simulink model "diff_drive_tracking_new"  (R2019b)
settings: Solver=ode45  StartTime=0.0  StopTime=T  MaxStep=0.01  RelTol=1e-3  EnableMultiTasking=on
values from neighbouring files (symbols this model uses):
  b = 1    [init.m]
  distc = 14.5    [init.m]
  radius = 3.25    [init.m]
  theta_0 = 0    [init.m]
  x_0 = 10    [init.m]
  y_0 = 40    [init.m]
undefined symbols (not defined in the file or in its folder): diff_drive, localization, potential
settings Model: ExtModeAutoUpdateStatusClock=off  Creator=marilena  LastModifiedBy=adelina
settings DataIOCC: LimitDataPoints=on  SaveFormat=Array  SignalLoggingSaveFormat=ModelDataLogs  ReturnWorkspaceOutputs=off
settings OptimizationCC: ExpressionDepthLimit=2147483647  LifeSpan=inf
settings DebuggingCC: SaveWithParameterizedLinksMsg=none  UnderspecifiedInitializationDetection=Classic  MergeDetectMultiDrivingBlocksExec=none  SolverPrmCheckMsg=warning  FcnCallInpInsideContextMsg=warning  StateNameClashWarn=warning  SFUnexpectedBacktrackingDiag=warning  SFNoUnconditionalDefaultTransitionDiag=warning  ArithmeticOperatorsInVariantConditions=warning
settings HardwareCC: ProdBitPerPointer=32  ProdBitPerSizeT=32  ProdBitPerPtrDiffT=32  ProdLargestAtomicFloat=None  ProdIntDivRoundTo=Undefined  ProdEndianess=Unspecified  ProdWordSize=32  ProdHWDeviceType=32-bit Generic  TargetHWDeviceType=32-bit Generic
settings ModelReferenceCC: PropagateSignalLabelsOutOfModel=off
settings SFSimCC: SimUseLocalCustomCode=off  CustomCodeUndefinedFunction=UseInterfaceOnly
settings RTWCC: RTWUseLocalCustomCode=off
settings CodeAppCC: StateflowObjectComments=on
settings GRTTargetCC: TargetFcnLib=ansi_tfl_tmw.mat  TargetLangStandard=C89/C90 (ANSI)  CombineOutputUpdateFcns=off  GRTInterface=on
settings ConfigComp: CovMetricSettings=dw  CovHtmlReporting=on  CovSaveCumulativeToWorkspaceVar=on  CovSaveSingleToWorkspaceVar=on  CovExternalEMLEnable=off

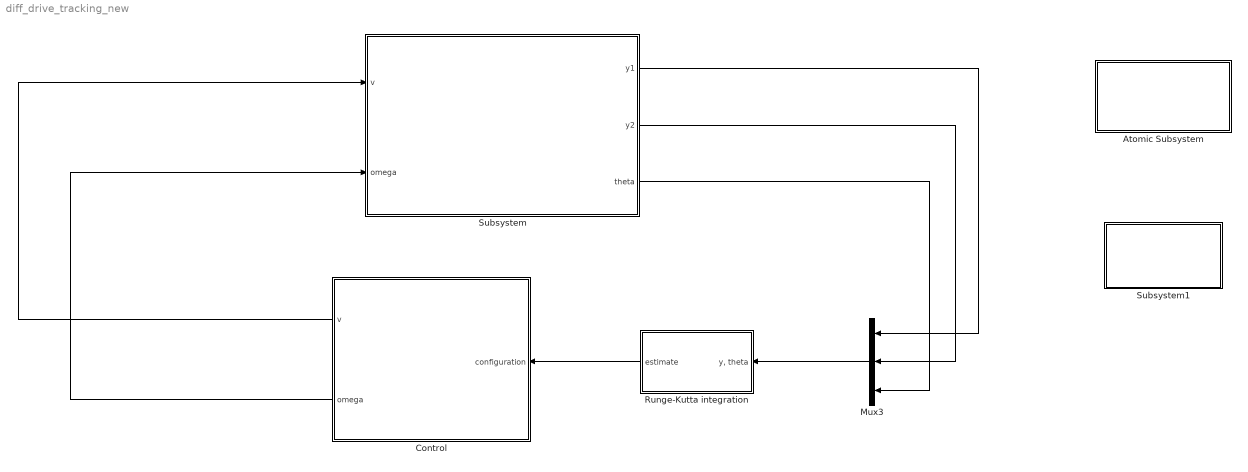
== system diff_drive_tracking_new ==
  Atomic Subsystem : Subsystem  TreatAsAtomicUnit=on
      settings: OpenFcn=init
      mask Display: disp('initialization')
  Control : Subsystem
  Mux3 : Mux  Inputs=3
  Runge-Kutta integration : Subsystem
  Subsystem : Subsystem
  Subsystem1 : Subsystem
      settings: OpenFcn=plots
      mask Display: disp('plots')
  wires:
  Mux3/1 -> Runge-Kutta integration/1("y, theta")
  Control/1(v) -> Subsystem/1(v)
  Control/2(omega) -> Subsystem/2(omega)
  Subsystem/1(y1) -> Mux3/1
  Subsystem/2(y2) -> Mux3/2
  Subsystem/3(theta) -> Mux3/3
  Runge-Kutta integration/1("estimate ") -> Control/1(configuration)

== system diff_drive_tracking_new/Atomic Subsystem ==

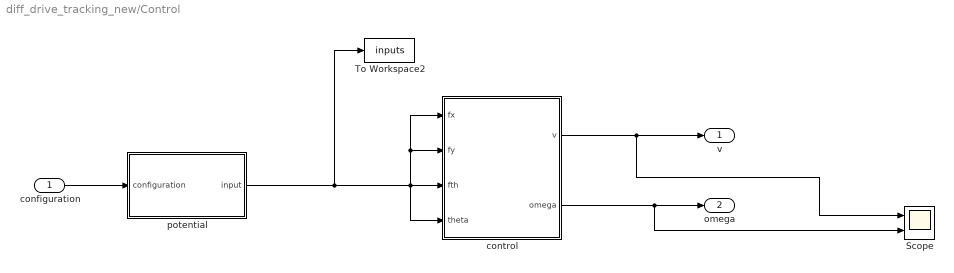
== system diff_drive_tracking_new/Control ==
  configuration : Inport
  Scope : Scope  NumInputPorts=2
  To Workspace2 : ToWorkspace  VariableName=inputs  SaveFormat=Structure With Time  SampleTime=-1
  control : Subsystem
  potential : Subsystem
  v : Outport
  omega : Outport  Port=2
  wires:
  control/2(omega) -> Scope/2, omega/1
  configuration/1 -> potential/1(configuration)
  potential/1(input) -> To Workspace2/1, control/1(fx), control/2(fy), control/4(theta), control/3(fth)
  control/1(v) -> Scope/1, v/1

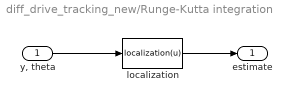
== system diff_drive_tracking_new/Runge-Kutta integration ==
  "y, theta" : Inport
  localization : MATLABFcn  Tag={'prova'}  Description=cartesian regulator  MATLABFcn=localization(u)  Output1D=off
  "estimate " : Outport  VectorParamsAs1DForOutWhenUnconnected=off
  wires:
  "y, theta"/1 -> localization/1
  localization/1 -> "estimate "/1

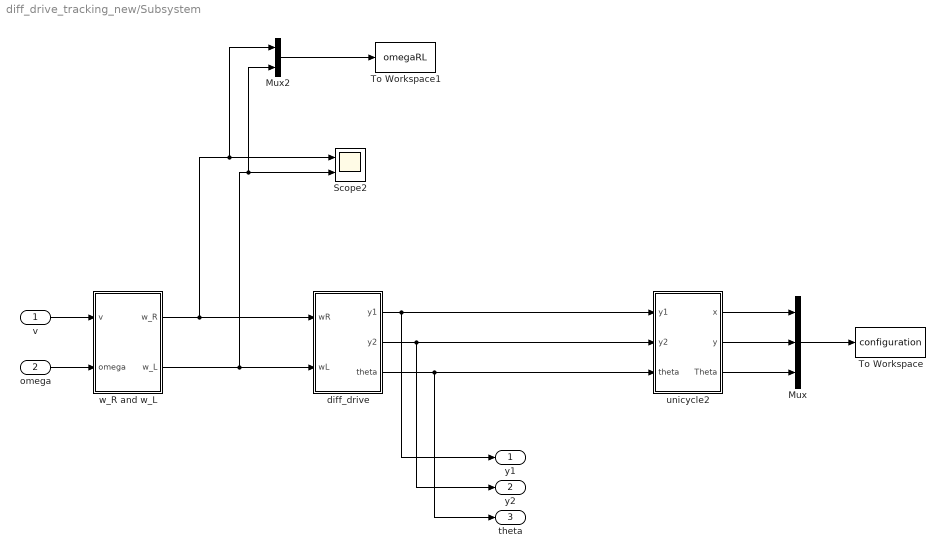
== system diff_drive_tracking_new/Subsystem ==
  v : Inport
  omega : Inport  Port=2
  Mux : Mux  Inputs=3
  Mux2 : Mux  Inputs=2
  Scope2 : Scope  NumInputPorts=2
  To Workspace : ToWorkspace  VariableName=configuration  SaveFormat=Structure With Time  SampleTime=-1
  To Workspace1 : ToWorkspace  VariableName=omegaRL  SaveFormat=Structure With Time  SampleTime=-1
  diff_drive : Subsystem
  unicycle2 : Subsystem
  "w_R and w_L " : Subsystem
  y1 : Outport
  y2 : Outport  Port=2
  theta : Outport  Port=3
  wires:
  unicycle2/3("Theta ") -> Mux/3
  unicycle2/1(x) -> Mux/1
  diff_drive/3(theta) -> theta/1, unicycle2/3(theta)
  Mux/1 -> To Workspace/1
  diff_drive/1(y1) -> y1/1, unicycle2/1(y1)
  diff_drive/2(y2) -> y2/1, unicycle2/2(y2)
  unicycle2/2(y) -> Mux/2
  v/1 -> "w_R and w_L "/1(v)
  "w_R and w_L "/2(w_L) -> Mux2/2, Scope2/2, diff_drive/2(wL)
  "w_R and w_L "/1(w_R) -> Mux2/1, Scope2/1, diff_drive/1(wR)
  Mux2/1 -> To Workspace1/1
  omega/1 -> "w_R and w_L "/2(omega)

== system diff_drive_tracking_new/Subsystem1 ==

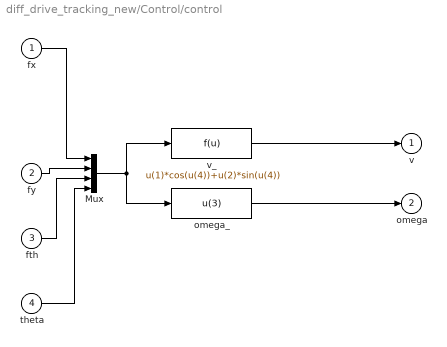
== system diff_drive_tracking_new/Control/control ==
  fx : Inport
  fy : Inport  Port=2
  fth : Inport  Port=3
  theta : Inport  Port=4
  Mux : Mux
  omega_ : Fcn  Expr=u(3)
  v_ : Fcn  Expr=u(1)*cos(u(4))+u(2)*sin(u(4))
  v : Outport  VectorParamsAs1DForOutWhenUnconnected=off
  omega : Outport  Port=2  VectorParamsAs1DForOutWhenUnconnected=off
  wires:
  fx/1 -> Mux/1
  fy/1 -> Mux/2
  v_/1 -> v/1
  omega_/1 -> omega/1
  Mux/1 -> v_/1, omega_/1
  fth/1 -> Mux/3
  theta/1 -> Mux/4

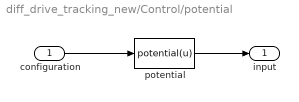
== system diff_drive_tracking_new/Control/potential ==
  configuration : Inport
  potential : MATLABFcn  Tag={'prova'}  Description=cartesian regulator  MATLABFcn=potential(u)  Output1D=off
  input : Outport  VectorParamsAs1DForOutWhenUnconnected=off
  wires:
  configuration/1 -> potential/1
  potential/1 -> input/1

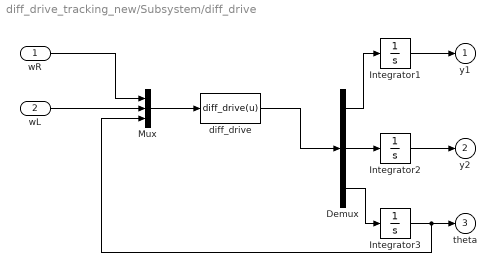
== system diff_drive_tracking_new/Subsystem/diff_drive ==
  wR : Inport
  wL : Inport  Port=2
  Demux : Demux  Outputs=3
  Integrator1 : Integrator  InitialCondition=x_0+b*cos(theta_0)
  Integrator2 : Integrator  InitialCondition=y_0+b*sin(theta_0)
  Integrator3 : Integrator  InitialCondition=theta_0
  Mux : Mux  Inputs=3
  diff_drive : MATLABFcn  Tag={'prova'}  Description=cartesian regulator  MATLABFcn=diff_drive(u)  Output1D=off
  y1 : Outport  VectorParamsAs1DForOutWhenUnconnected=off
  y2 : Outport  Port=2  VectorParamsAs1DForOutWhenUnconnected=off
  theta : Outport  Port=3  VectorParamsAs1DForOutWhenUnconnected=off
  wires:
  wR/1 -> Mux/1
  wL/1 -> Mux/2
  Mux/1 -> diff_drive/1
  diff_drive/1 -> Demux/1
  Demux/1 -> Integrator1/1
  Integrator1/1 -> y1/1
  Demux/2 -> Integrator2/1
  Integrator2/1 -> y2/1
  Demux/3 -> Integrator3/1
  Integrator3/1 -> Mux/3, theta/1

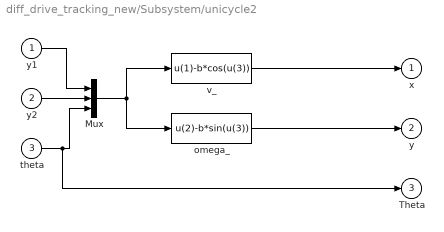
== system diff_drive_tracking_new/Subsystem/unicycle2 ==
  y1 : Inport
  y2 : Inport  Port=2
  theta : Inport  Port=3
  Mux : Mux  Inputs=3
  omega_ : Fcn  Expr=u(2)-b*sin(u(3))
  v_ : Fcn  Expr=u(1)-b*cos(u(3))
  x : Outport  VectorParamsAs1DForOutWhenUnconnected=off
  y : Outport  Port=2  VectorParamsAs1DForOutWhenUnconnected=off
  "Theta " : Outport  Port=3  VectorParamsAs1DForOutWhenUnconnected=off
  wires:
  y1/1 -> Mux/1
  y2/1 -> Mux/2
  v_/1 -> x/1
  omega_/1 -> y/1
  Mux/1 -> v_/1, omega_/1
  theta/1 -> "Theta "/1, Mux/3

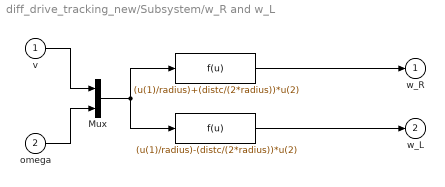
== system diff_drive_tracking_new/Subsystem/w_R and w_L  ==
  v : Inport
  omega : Inport  Port=2
  " " : Fcn  Expr=(u(1)/radius)+(distc/(2*radius))*u(2)
  " " : Fcn  Expr=(u(1)/radius)-(distc/(2*radius))*u(2)
  Mux : Mux  Inputs=2
  w_R : Outport  VectorParamsAs1DForOutWhenUnconnected=off
  w_L : Outport  Port=2  VectorParamsAs1DForOutWhenUnconnected=off
  wires:
  v/1 -> Mux/1
  omega/1 -> Mux/2
  " "/1 -> w_R/1
  " "/1 -> w_L/1
  Mux/1 -> " "/1, " "/1
